simulink model "ADC"  (R2021a)
settings: Solver=VariableStepAuto  StartTime=0.0  StopTime=Inf  RelTol=1e-3
libraries: commdigbbndam3 x2, dspsigops x2, dspquant2 x2, commchan3 x1, commsink2 x1
settings Model: Creator=Bharat Gunhalkar  LastModifiedBy=Bharat Gunhalkar

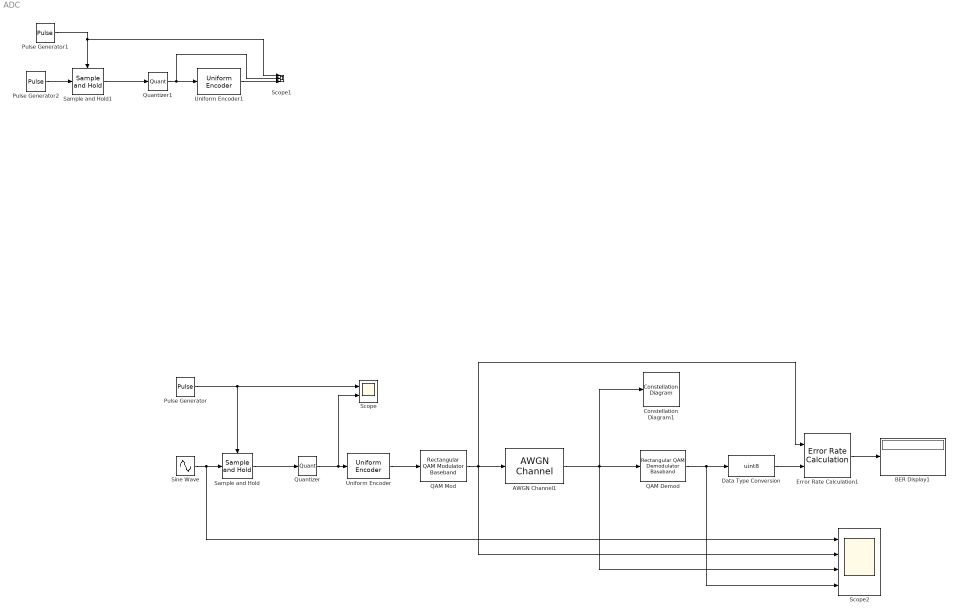
== system ADC ==
  AWGN Channel1 : commchan3/AWGN Channel  InputProcessing=Columns as channels (frame based)  seed=67  noiseMode="Signal to noise ratio  (Eb/No)"  EbNodB=1  EsNodB=10  SNRdB=10  bitsPerSym=1  Ps=1  Tsym=1  variance=1
  BER Display1 : Display
  Constellation Diagram1 : ConstellationDiagram
  Data Type Conversion : DataTypeConversion  OutDataTypeStr=uint8
  Error Rate Calculation1 : commsink2/Error Rate Calculation  N=0  st_delay=0  cp_mode=Entire frame  subframe=[]  PMode=Port  WsName=ErrorVec  RsMode2=off  stop=off  numErr=100  maxBits=1e6
  Pulse Generator : DiscretePulseGenerator  Period=1000  PulseWidth=5
  Pulse Generator1 : DiscretePulseGenerator  PulseType=Time based  Period=.001  PulseWidth=5
  Pulse Generator2 : DiscretePulseGenerator  PulseType=Time based  Amplitude=8  Period=1  PulseWidth=30
  QAM Demod : commdigbbndam3/Rectangular QAM Demodulator Baseband  M=16  OutType=Integer  DecType=Hard decision  VarSource=Dialog  Variance=1  Dec=Gray  Mapping=[0:15]  PowType=Min. distance between symbols  MinDist=2  AvgPow=1  PeakPow=1  Ph=0  outDtype1=Inherit via internal rule  outDtype2=Inherit via internal rule  derotateFactorWordLen=16  derotateFactorDataTypeStr=Inherit: Same word length as input  derotateFactorLastDataTypeStr=Inherit: Same word length as input  denormFactorWordLen=16  denormFactorDataTypeStr=Inherit: Same word length as input  denormFactorLastDataTypeStr=Inherit: Same word length as input  prodOutWordLen=32  prodOutOverflowMode=Wrap  prodOutRoundingMode=Floor  prodOutOvFlMode=off  prodOutOvFlModeLastStrValue=off  sumWordLen=32
  QAM Mod : commdigbbndam3/Rectangular QAM Modulator Baseband  M=16  InType=Integer  Enc=Gray  Mapping=[0:15]  PowType=Min. distance between symbols  MinDist=2  AvgPow=1  PeakPow=1  Ph=0  outDtype=double  outWordLen=16  outUDDataType=sfix(16)  outFracLenMode=Best precision  outFracLen=15  outDataTypeStr=double  outLastDataTypeStr=double
  Quantizer : Quantizer  QuantizationInterval=0.25  LinearizeAsGain=off
  Quantizer1 : Quantizer  QuantizationInterval=0.125  LinearizeAsGain=off
  Sample and Hold : dspsigops/Sample and Hold  trig=Rising edge  initCond=0  latchinput=off
  Sample and Hold1 : dspsigops/Sample and Hold  trig=Rising edge  initCond=0  latchinput=off
  Scope : Scope  NumInputPorts=2
  Scope1 : Scope  NumInputPorts=3
  Scope2 : Scope  NumInputPorts=4
  Sine Wave : Sin  Amplitude=10  SampleTime=0
  Uniform Encoder : dspquant2/Uniform Encoder  peak=1  bits=4  otype=Unsigned integer
  Uniform Encoder1 : dspquant2/Uniform Encoder  peak=1  bits=8  otype=Unsigned integer
  wires:
  Sine Wave/1 -> Scope2/1, Sample and Hold/1
  Pulse Generator/1 -> Sample and Hold/Trigger, Scope/1
  Sample and Hold/1 -> Quantizer/1
  Quantizer/1 -> Scope/2, Uniform Encoder/1
  Quantizer1/1 -> Scope1/2, Uniform Encoder1/1
  Pulse Generator1/1 -> Sample and Hold1/Trigger, Scope1/1
  Sample and Hold1/1 -> Quantizer1/1
  Pulse Generator2/1 -> Sample and Hold1/1
  Uniform Encoder1/1 -> Scope1/3
  Error Rate Calculation1/1 -> BER Display1/1
  QAM Demod/1 -> Scope2/4, Data Type Conversion/1
  QAM Mod/1 -> Scope2/2, Error Rate Calculation1/1, AWGN Channel1/1
  AWGN Channel1/1 -> Scope2/3, QAM Demod/1, Constellation Diagram1/1
  Data Type Conversion/1 -> Error Rate Calculation1/2
  Uniform Encoder/1 -> QAM Mod/1
